simulink model "model_from_encoders"  (R2018a)
settings: Solver=VariableStepAuto  StartTime=0.0  StopTime=100  MaxStep=0.01  RelTol=1e-3
libraries: robotcorelib x1, simulink x1
settings Model: Creator=S  LastModifiedBy=reiserbalazs

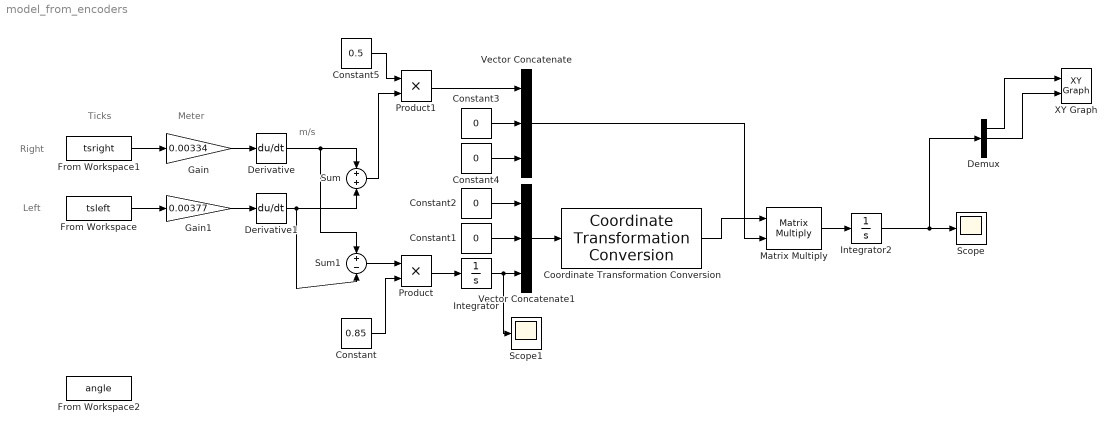
== system model_from_encoders ==
  note: Right
  note: Left
  note: m/s
  note: Meter
  note: Ticks
  Constant : Constant  Value=0.85
  Constant{1..4} (4 alike) : Constant  Value=0
  Constant5 : Constant  Value=0.5
  Coordinate Transformation Conversion : robotcorelib/Coordinate Transformation Conversion  InputRepresentation=Euler Angles  InputEulerSequence=XYZ  ShowTrVecInputPort=on  OutputRepresentation=Rotation Matrix  OutputEulerSequence=ZYX  ShowTrVecOutputPort=on  SimulateUsing=Interpreted execution
      settings: SourceProductBaseCode=RO
  Demux : Demux  Outputs=3
  Derivative : Derivative
  Derivative1 : Derivative
  From Workspace : FromWorkspace  VariableName=tsleft  SampleTime=0
  From Workspace1 : FromWorkspace  VariableName=tsright  SampleTime=0
  From Workspace2 : FromWorkspace  VariableName=angle  SampleTime=0
  Gain : Gain  Gain=0.00334
  Gain1 : Gain  Gain=0.00377
  Integrator : Integrator
  Integrator2 : Integrator
  Matrix Multiply : Product  Multiplication=Matrix(*)
  Product : Product
  Product1 : Product
  Scope : Scope
  Scope1 : Scope
  Sum : Sum  Inputs=+|+
  Sum1 : Sum  Inputs=+|-
  Vector Concatenate : Concatenate  NumInputs=3
  Vector Concatenate1 : Concatenate  NumInputs=3
  XY Graph : simulink/Sinks/XY Graph  xmin=-300  xmax=300  ymin=-300  ymax=300  st=-1
  wires:
  Derivative/1 -> Sum1/1, Sum/1
  Derivative1/1 -> Sum1/2, Sum/2
  Sum1/1 -> Product/1
  Product/1 -> Integrator/1
  Constant/1 -> Product/2
  Integrator/1 -> Scope1/1, Vector Concatenate1/3
  Sum/1 -> Product1/2
  Constant2/1 -> Vector Concatenate1/1
  Constant1/1 -> Vector Concatenate1/2
  Constant3/1 -> Vector Concatenate/2
  Constant4/1 -> Vector Concatenate/3
  Vector Concatenate1/1 -> Coordinate Transformation Conversion/1
  Integrator2/1 -> Demux/1, Scope/1
  Matrix Multiply/1 -> Integrator2/1
  Coordinate Transformation Conversion/1 -> Matrix Multiply/1
  Product1/1 -> Vector Concatenate/1
  Constant5/1 -> Product1/1
  Gain/1 -> Derivative/1
  Gain1/1 -> Derivative1/1
  Vector Concatenate/1 -> Matrix Multiply/2
  From Workspace/1 -> Gain1/1
  From Workspace1/1 -> Gain/1
  Demux/1 -> XY Graph/1
  Demux/2 -> XY Graph/2
